simulink model "Wing_Model_SAAM"  (R2018a)
settings: Solver=FixedStepAuto  StartTime=0.0  StopTime=10.0  FixedStep=dt  RelTol=1e-3
values from neighbouring files (symbols this model uses):
  Aw = 4.6    [airplane_ic_constants.m]
  CD0_w = 0.01    [airplane_ic_constants.m]
  CDfp_w = 1    [airplane_ic_constants.m]
  CL0_w = 0    [airplane_ic_constants.m]
  CLmax_w = 1.1    [airplane_ic_constants.m]
  Kw = 0.060    (= 0.06)    [airplane_ic_constants.m]
  S = 13.0    (= 13)    [airplane_ic_constants.m]
  tauAil = 0.4    [airplane_ic_constants.m]
libraries: simulink x3
settings Model: Creator=Kyle  LastModifiedBy=Kyle

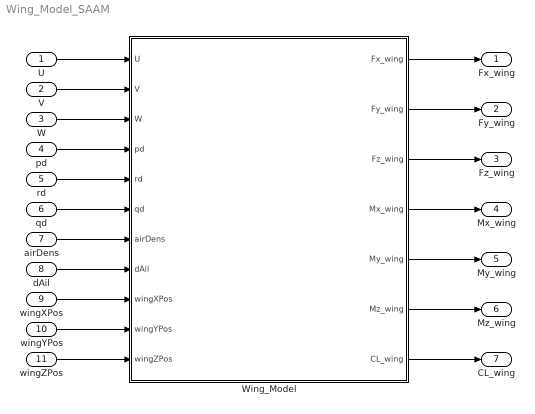
== system Wing_Model_SAAM ==
  U : Inport
  V : Inport  Port=2
  W : Inport  Port=3
  pd : Inport  Port=4
  rd : Inport  Port=5
  qd : Inport  Port=6
  airDens : Inport  Port=7
  dAil : Inport  Port=8
  wingXPos : Inport  Port=9
  wingYPos : Inport  Port=10
  wingZPos : Inport  Port=11
  Wing_Model : Subsystem
  Fx_wing : Outport
  Fy_wing : Outport  Port=2
  Fz_wing : Outport  Port=3
  Mx_wing : Outport  Port=4
  My_wing : Outport  Port=5
  Mz_wing : Outport  Port=6
  CL_wing : Outport  Port=7
  wires:
  U/1 -> Wing_Model/1(U)
  V/1 -> Wing_Model/2(V)
  W/1 -> Wing_Model/3(W)
  pd/1 -> Wing_Model/4(pd)
  wingXPos/1 -> Wing_Model/9(wingXPos)
  wingYPos/1 -> Wing_Model/10(wingYPos)
  wingZPos/1 -> Wing_Model/11(wingZPos)
  dAil/1 -> Wing_Model/8(dAil)
  rd/1 -> Wing_Model/5(rd)
  qd/1 -> Wing_Model/6(qd)
  airDens/1 -> Wing_Model/7(airDens)
  Wing_Model/4(Mx_wing) -> Mx_wing/1
  Wing_Model/6(Mz_wing) -> Mz_wing/1
  Wing_Model/5(My_wing) -> My_wing/1
  Wing_Model/2(Fy_wing) -> Fy_wing/1
  Wing_Model/1(Fx_wing) -> Fx_wing/1
  Wing_Model/3(Fz_wing) -> Fz_wing/1
  Wing_Model/7(CL_wing) -> CL_wing/1

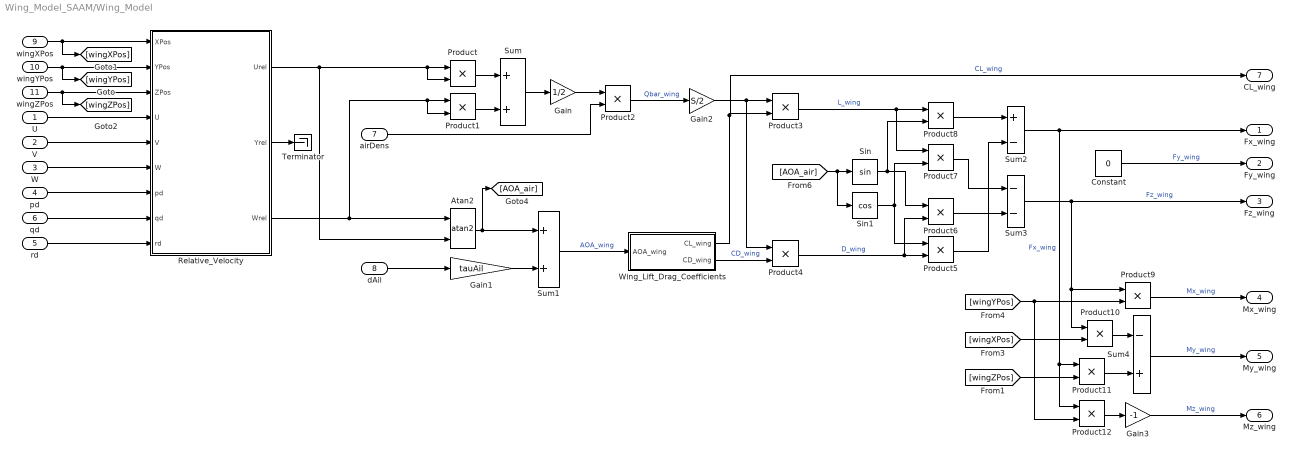
== system Wing_Model_SAAM/Wing_Model ==
  U : Inport
  V : Inport  Port=2
  W : Inport  Port=3
  pd : Inport  Port=4
  rd : Inport  Port=5
  qd : Inport  Port=6
  airDens : Inport  Port=7
  dAil : Inport  Port=8
  wingXPos : Inport  Port=9
  wingYPos : Inport  Port=10
  wingZPos : Inport  Port=11
  Atan2 : Trigonometry  Operator=atan2
  Constant : Constant  Value=0
  Gain : Gain  Gain=1/2
  Gain1 : Gain  Gain=tauAil
  Gain2 : Gain  Gain=S/2
  Gain3 : Gain  Gain=-1
  Product{,1..12} (13 alike) : Product
  Relative_Velocity : Subsystem
  Sin : Trigonometry
  Sin1 : Trigonometry  Operator=cos
  Sum : Sum
  Sum1 : Sum
  Sum2 : Sum  Inputs=+-
  Sum3 : Sum  Inputs=--
  Sum4 : Sum  Inputs=-+
  Terminator : Terminator
  Wing_Lift_Drag_Coefficients : Subsystem
  Fx_wing : Outport
  Fy_wing : Outport  Port=2
  Fz_wing : Outport  Port=3
  Mx_wing : Outport  Port=4
  My_wing : Outport  Port=5
  Mz_wing : Outport  Port=6
  CL_wing : Outport  Port=7
  wires:
  wingYPos/1 -> [wingYPos], Relative_Velocity/2(YPos)
  wingZPos/1 -> [wingZPos], Relative_Velocity/3(ZPos)
  U/1 -> Relative_Velocity/4(U)
  V/1 -> Relative_Velocity/5(V)
  W/1 -> Relative_Velocity/6(W)
  pd/1 -> Relative_Velocity/7(pd)
  rd/1 -> Relative_Velocity/9(rd)
  qd/1 -> Relative_Velocity/8(qd)
  Relative_Velocity/3(Wrel) -> Product1/2, Product1/1, Atan2/1
  Sum/1 -> Gain/1
  Product/1 -> Sum/1
  Product1/1 -> Sum/2
  Gain/1 -> Product2/1
  airDens/1 -> Product2/2
  Relative_Velocity/1(Urel) -> Atan2/2, Product/2, Product/1
  dAil/1 -> Gain1/1
  Gain1/1 -> Sum1/2
  Atan2/1 -> [AOA_air], Sum1/1
  Product2/1 -> Gain2/1  "Qbar_wing"
  Sum1/1 -> Wing_Lift_Drag_Coefficients/1(AOA_wing)  "AOA_wing"
  Gain2/1 -> Product4/1, Product3/1
  Wing_Lift_Drag_Coefficients/1(CL_wing) -> CL_wing/1, Product3/2  "CL_wing"
  Wing_Lift_Drag_Coefficients/2("CD_wing ") -> Product4/2  "CD_wing"
  Product4/1 -> Product5/2, Product6/2  "D_wing"
  [AOA_air] -> Sin1/1, Sin/1
  Sin1/1 -> Product5/1, Product7/2
  Sin/1 -> Product8/2, Product6/1
  Product3/1 -> Product7/1, Product8/1  "L_wing"
  Product8/1 -> Sum2/1
  Product5/1 -> Sum2/2
  Product7/1 -> Sum3/1
  Product6/1 -> Sum3/2
  Sum3/1 -> Fz_wing/1, Product9/1, Product10/1  "Fz_wing"
  Constant/1 -> Fy_wing/1  "Fy_wing"
  wingXPos/1 -> [wingXPos], Relative_Velocity/1(XPos)
  [wingYPos] -> Product12/2, Product9/2
  Product9/1 -> Mx_wing/1  "Mx_wing"
  Sum2/1 -> Product12/1, Product11/1, Fx_wing/1  "Fx_wing"
  [wingXPos] -> Product10/2
  [wingZPos] -> Product11/2
  Product10/1 -> Sum4/1
  Product11/1 -> Sum4/2
  Sum4/1 -> My_wing/1  "My_wing"
  Product12/1 -> Gain3/1
  Gain3/1 -> Mz_wing/1  "Mz_wing"
  Relative_Velocity/2(Yrel) -> Terminator/1

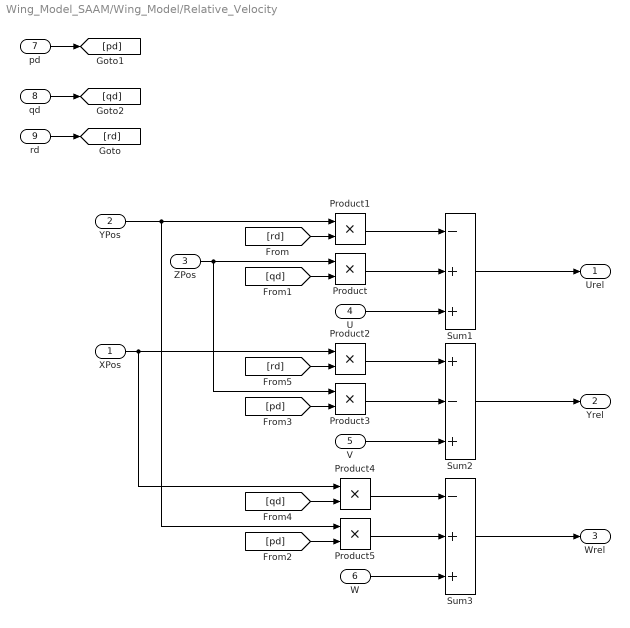
== system Wing_Model_SAAM/Wing_Model/Relative_Velocity ==
  XPos : Inport
  YPos : Inport  Port=2
  ZPos : Inport  Port=3
  U : Inport  Port=4
  V : Inport  Port=5
  W : Inport  Port=6
  pd : Inport  Port=7
  qd : Inport  Port=8
  rd : Inport  Port=9
  Product{,1..5} (6 alike) : Product
  Sum1 : Sum  Inputs=-++
  Sum2 : Sum  Inputs=+-+
  Sum3 : Sum  Inputs=-++
  Urel : Outport
  Yrel : Outport  Port=2
  Wrel : Outport  Port=3
  wires:
  ZPos/1 -> Product3/1, Product/1
  Product/1 -> Sum1/2
  U/1 -> Sum1/3
  [rd] -> Product1/2
  Product1/1 -> Sum1/1
  rd/1 -> [rd]
  Sum1/1 -> Urel/1
  pd/1 -> [pd]
  qd/1 -> [qd]
  [qd] -> Product/2
  V/1 -> Sum2/3
  Sum2/1 -> Yrel/1
  Sum3/1 -> Wrel/1
  W/1 -> Sum3/3
  Product3/1 -> Sum2/2
  Product2/1 -> Sum2/1
  XPos/1 -> Product4/1, Product2/1
  YPos/1 -> Product5/1, Product1/1
  Product5/1 -> Sum3/2
  Product4/1 -> Sum3/1
  [pd] -> Product5/2
  [pd] -> Product3/2
  [rd] -> Product2/2
  [qd] -> Product4/2

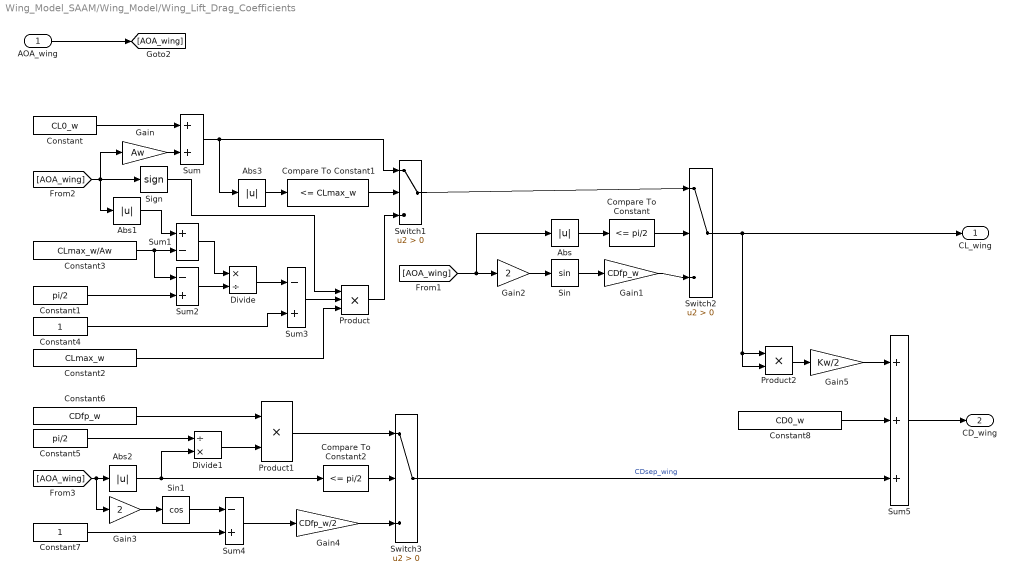
== system Wing_Model_SAAM/Wing_Model/Wing_Lift_Drag_Coefficients ==
  AOA_wing : Inport
  Abs{,1..3} (4 alike) : Abs
  Compare To Constant : simulink/Logic and Bit Operations/Compare To Constant  relop=<=  const=pi/2  OutDataTypeStr=boolean
  Compare To Constant1 : simulink/Logic and Bit Operations/Compare To Constant  relop=<=  const=CLmax_w  OutDataTypeStr=boolean
  Compare To Constant2 : simulink/Logic and Bit Operations/Compare To Constant  relop=<=  const=pi/2  OutDataTypeStr=boolean
  Constant : Constant  Value=CL0_w
  Constant1 : Constant  Value=pi/2
  Constant2 : Constant  Value=CLmax_w
  Constant3 : Constant  Value=CLmax_w/Aw
  Constant4 : Constant
  Constant5 : Constant  Value=pi/2
  Constant6 : Constant  Value=CDfp_w
  Constant7 : Constant
  Constant8 : Constant  Value=CD0_w
  Divide : Product  Inputs=*/
  Divide1 : Product  Inputs=/*
  Gain : Gain  Gain=Aw
  Gain1 : Gain  Gain=CDfp_w
  Gain2 : Gain  Gain=2
  Gain3 : Gain  Gain=2
  Gain4 : Gain  Gain=CDfp_w/2
  Gain5 : Gain  Gain=Kw/2
  Product : Product  Inputs=3
  Product1 : Product
  Product2 : Product
  Sign : Signum
  Sin : Trigonometry
  Sin1 : Trigonometry  Operator=cos
  Sum : Sum
  Sum1 : Sum  Inputs=+-
  Sum2 : Sum  Inputs=-+
  Sum3 : Sum  Inputs=-+
  Sum4 : Sum  Inputs=-+
  Sum5 : Sum  Inputs=+++
  Switch1 : Switch  Criteria=u2 > Threshold
  Switch2 : Switch  Criteria=u2 > Threshold
  Switch3 : Switch  Criteria=u2 > Threshold
  CL_wing : Outport
  "CD_wing " : Outport  Port=2
  wires:
  Compare To Constant/1 -> Switch2/2
  AOA_wing/1 -> [AOA_wing]
  [AOA_wing] -> Gain2/1, Abs/1
  Abs/1 -> Compare To Constant/1
  Abs1/1 -> Sum1/1
  [AOA_wing] -> Sign/1, Abs1/1, Gain/1
  Compare To Constant1/1 -> Switch1/2
  Constant/1 -> Sum/1
  Gain/1 -> Sum/2
  Sum/1 -> Abs3/1, Switch1/1
  Constant3/1 -> Sum2/1, Sum1/2
  Constant1/1 -> Sum2/2
  Sum1/1 -> Divide/1
  Sum2/1 -> Divide/2
  Constant4/1 -> Sum3/2
  Divide/1 -> Sum3/1
  Sum3/1 -> Product/2
  Constant2/1 -> Product/3
  Product/1 -> Switch1/3
  Switch1/1 -> Switch2/1
  Gain1/1 -> Switch2/3
  Switch2/1 -> CL_wing/1, Product2/1, Product2/2
  Sin/1 -> Gain1/1
  Gain2/1 -> Sin/1
  [AOA_wing] -> Gain3/1, Abs2/1
  Compare To Constant2/1 -> Switch3/2
  Abs2/1 -> Compare To Constant2/1, Divide1/2
  Constant5/1 -> Divide1/1
  Divide1/1 -> Product1/2
  Product1/1 -> Switch3/1
  Constant6/1 -> Product1/1
  Sin1/1 -> Sum4/1
  Gain3/1 -> Sin1/1
  Constant7/1 -> Sum4/2
  Sum4/1 -> Gain4/1
  Gain4/1 -> Switch3/3
  Switch3/1 -> Sum5/3  "CDsep_wing"
  Product2/1 -> Gain5/1
  Gain5/1 -> Sum5/1
  Sum5/1 -> "CD_wing "/1
  Constant8/1 -> Sum5/2
  Abs3/1 -> Compare To Constant1/1
  Sign/1 -> Product/1
